simulink model "ForEach4"  (R2017b)
settings: Solver=FixedStepDiscrete  StartTime=0.0  StopTime=10.0  FixedStep=0.200000  RelTol=1e-3  EnableMultiTasking=on
settings Model: Creator=hbourbou  LastModifiedBy=hbourbou
settings DataIOCC: LimitDataPoints=on  SaveFormat=Structure
settings OptimizationCC: LifeSpan=inf
settings DebuggingCC: SFUnexpectedBacktrackingDiag=warning  SFNoUnconditionalDefaultTransitionDiag=warning  SFExecutionAtInitializationDiag=none
settings HardwareCC: ProdBitPerPointer=32  ProdBitPerSizeT=32  ProdBitPerPtrDiffT=32  ProdLargestAtomicFloat=None  ProdIntDivRoundTo=Undefined  ProdEndianess=Unspecified  ProdWordSize=32  ProdHWDeviceType=32-bit Generic
settings ModelReferenceCC: PropagateSignalLabelsOutOfModel=off
settings CodeAppCC: StateflowObjectComments=on
settings GRTTargetCC: TargetLangStandard=C89/C90 (ANSI)  GeneratePreprocessorConditionals=Disable all
settings ConfigComp: CovMetricSettings=dw  CovHtmlReporting=on  CovSaveCumulativeToWorkspaceVar=on  CovSaveSingleToWorkspaceVar=on  CovExternalEMLEnable=off

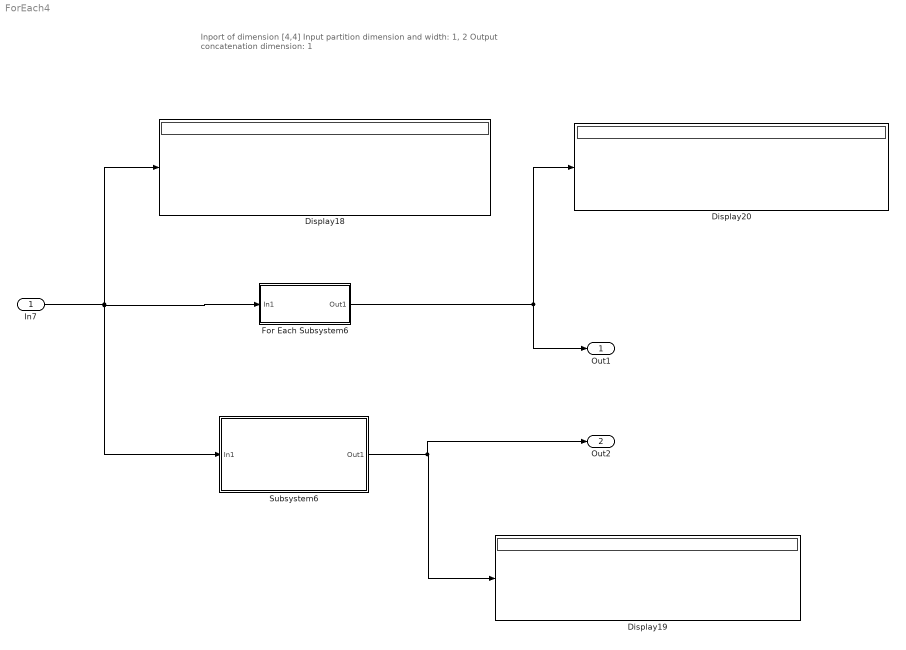
== system ForEach4 ==
  note: Inport of dimension [4,4]
      | Input partition dimension and width: 1, 2
      | Output concatenation dimension: 1
  In7 : Inport  PortDimensions=[4 4]
  Display18 : Display
  Display19 : Display
  Display20 : Display
  For Each Subsystem6 : Subsystem
  Subsystem6 : Subsystem
  Out1 : Outport
  Out2 : Outport  Port=2
  wires:
  In7/1 -> For Each Subsystem6/1(In1), Subsystem6/1(In1), Display18/1
  For Each Subsystem6/1(Out1) -> Display20/1, Out1/1
  Subsystem6/1(Out1) -> Out2/1, Display19/1

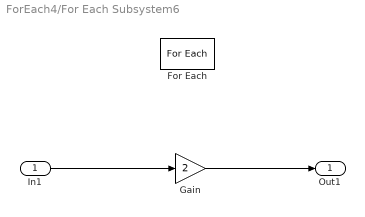
== system ForEach4/For Each Subsystem6 ==
  In1 : Inport  Partition=on  PartitionDimension=1  PartitionWidth=2  PartitionOffset=0
  For Each : ForEach  DisableCoverage=on  IndexMode=One-based
  Gain : Gain  Gain=2
  Out1 : Outport  ConcatenationDimension=1
  wires:
  Gain/1 -> Out1/1
  In1/1 -> Gain/1

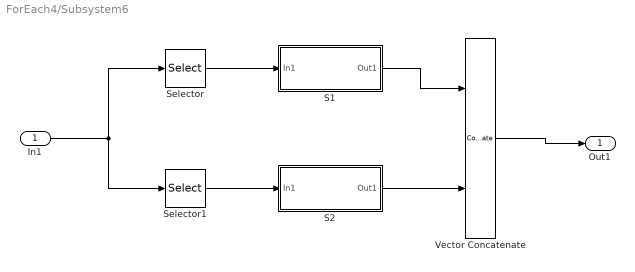
== system ForEach4/Subsystem6 ==
  In1 : Inport
  S1 : Subsystem
  S2 : Subsystem
  Selector : Selector  NumberOfDimensions=2  InputPortWidth=3  IndexOptions=Index vector (dialog),Select all  Indices=[1 2],  OutputSizes=1,1
  Selector1 : Selector  NumberOfDimensions=2  InputPortWidth=3  IndexOptions=Index vector (dialog),Select all  Indices=[3 4],  OutputSizes=1,1
  Vector Concatenate : Concatenate  Mode=Multidimensional array
  Out1 : Outport
  wires:
  S1/1(Out1) -> Vector Concatenate/1
  S2/1(Out1) -> Vector Concatenate/2
  Selector/1 -> S1/1(In1)
  Vector Concatenate/1 -> Out1/1
  Selector1/1 -> S2/1(In1)
  In1/1 -> Selector1/1, Selector/1

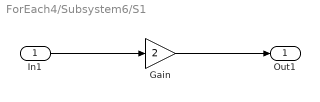
== system ForEach4/Subsystem6/S1 ==
  In1 : Inport
  Gain : Gain  Gain=2
  Out1 : Outport
  wires:
  In1/1 -> Gain/1
  Gain/1 -> Out1/1

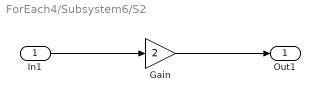
== system ForEach4/Subsystem6/S2 ==
  In1 : Inport
  Gain : Gain  Gain=2
  Out1 : Outport
  wires:
  In1/1 -> Gain/1
  Gain/1 -> Out1/1
